simulink model "motor"  (Simulink 3.00)
libraries: mathlib x62, logiclib x16, reglib x10, execlib x6, genlib x6, anallib x4, arclib x1

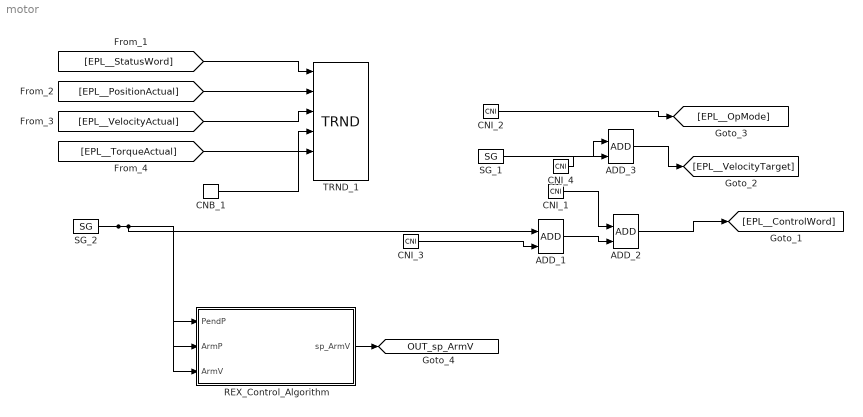
== system motor ==
  ADD_1 : mathlib/ADD
  ADD_2 : mathlib/ADD
  ADD_3 : mathlib/ADD
  CNB_1 : mathlib/CNB  YCN=on
  CNI_1 : mathlib/CNI  icn=15
  CNI_2 : mathlib/CNI  icn=3
  CNI_3 : mathlib/CNI  icn=64
  CNI_4 : mathlib/CNI  icn=0
  REX_Control_Algorithm : Subsystem  TreatAsAtomicUnit=on  SystemSampleTime=0.003
      mask Type: REX sequence
  SG_1 : genlib/SG  isig=1: SINE  amp=3000  freq=0.05  phase=0  ifrunit=1: Hz  iphunit=1: degree
  SG_2 : genlib/SG  isig=2: SQUARE  amp=64  freq=0.1  phase=0  ifrunit=1: Hz  iphunit=1: degree
  TRND_1 : arclib/TRND  n=4  l=1000  btype=8: Double  ptype1=1: Store  ptype2=1: Store  ptype3=1: Store  ptype4=1: Store  pfac=1  afac=0  arc=0  id=1  Title=Trend Title
  tag scope: OUT_sp_ArmV=global
  wires:
  ADD_1/1 -> ADD_2/2
  ADD_2/1 -> [EPL__ControlWord]
  ADD_3/1 -> [EPL__VelocityTarget]
  CNB_1/1 -> TRND_1/5
  CNI_1/1 -> ADD_2/1
  CNI_2/1 -> [EPL__OpMode]
  CNI_3/1 -> ADD_1/2
  CNI_4/1 -> ADD_3/2
  [EPL__StatusWord] -> TRND_1/1
  [EPL__PositionActual] -> TRND_1/2
  [EPL__VelocityActual] -> TRND_1/3
  [EPL__TorqueActual] -> TRND_1/4
  REX_Control_Algorithm/1(sp_ArmV) -> [OUT_sp_ArmV]
  SG_1/1 -> ADD_3/1
  SG_2/1 -> REX_Control_Algorithm/1(PendP), REX_Control_Algorithm/2(ArmP), ADD_1/1, REX_Control_Algorithm/3(ArmV)

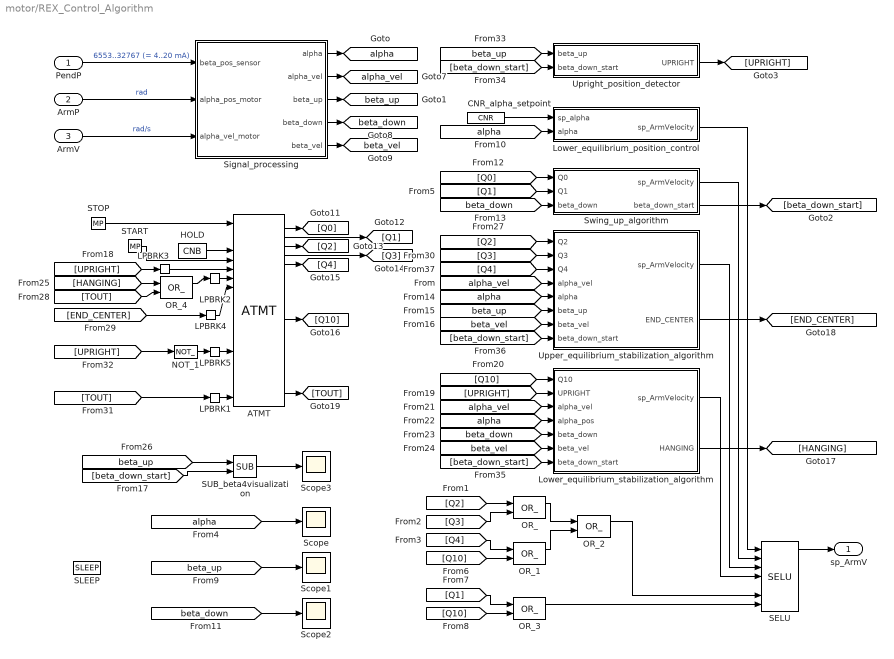
== system motor/REX_Control_Algorithm ==
  PendP : Inport  Port=1
  ArmP : Inport  Port=2
  ArmV : Inport  Port=3
  ATMT : logiclib/ATMT  SystemSampleTime=-1  morestps=off  ntr=10  STT=[0 0 1;1 1 2;1 15 0;2 3 3;3 15 4;4 15 10;10 2 0;2 10 0;3 10 0;4 10 0]  touts=[100 1 20 10 10 0 0 0 0 0 5 0 0 0 0 0]
  CNR_alpha_setpoint : mathlib/CNR  SystemSampleTime=-1  ycn=0
  HOLD : mathlib/CNB  SystemSampleTime=-1  YCN=off
  LPBRK{1..5} (5 alike) : execlib/LPBRK
  Lower_equilibrium_position_control : Subsystem
      mask Type: REX sequence
  Lower_equilibrium_stabilization_algorithm : Subsystem
      mask Type: REX sequence
  NOT_1 : logiclib/NOT_  SystemSampleTime=-1
  OR_{,1..4} (5 alike) : logiclib/OR_  SystemSampleTime=-1
  SELU : reglib/SELU  SystemSampleTime=-1  BINF=on
  SLEEP : execlib/SLEEP  SystemSampleTime=-1  ts=0.01
  START : genlib/MP  SystemSampleTime=-1  pwidth=0.01  BSTATE=off  RPTF=off
  STOP : genlib/MP  SystemSampleTime=-1  pwidth=0.01  BSTATE=off  RPTF=off
  SUB_beta4visualization : mathlib/SUB  SystemSampleTime=-1
  Scope{,1..3} (4 alike) : Scope
      Scope settings: TimeRange=60  YMin=-4  YMax=2
      Scope1 settings: TimeRange=60  YMin=-4  YMax=4
      Scope2 settings: YMin=2.97087  YMax=2.97104  SaveName=ScopeData2
      Scope3 settings: YMin=0  YMax=3.25  SaveName=ScopeData4
  Signal_processing : Subsystem
      mask Type: REX sequence
  Swing_up_algorithm : Subsystem
      mask Type: REX sequence
  Upper_equilibrium_stabilization_algorithm : Subsystem
      mask Type: REX sequence
  Upright_position_detector : Subsystem
      mask Type: REX sequence
  sp_ArmV : Outport  Port=1
  tag scope: alpha=global, alpha_vel=global, beta_down=global, beta_up=global, beta_vel=global
  wires:
  ATMT/1 -> [Q0]
  ATMT/2 -> [Q1]
  ATMT/3 -> [Q2]
  ATMT/4 -> [Q3]
  ATMT/5 -> [Q4]
  ATMT/11 -> [Q10]
  ATMT/19 -> [TOUT]
  ArmP/1 -> Signal_processing/2(alpha_pos_motor)  "rad"
  ArmV/1 -> Signal_processing/3(alpha_vel_motor)  "rad/s"
  CNR_alpha_setpoint/1 -> Lower_equilibrium_position_control/1(sp_alpha)
  [alpha_vel] -> Upper_equilibrium_stabilization_algorithm/4(alpha_vel)
  [Q2] -> OR_/1
  [alpha] -> Lower_equilibrium_position_control/2(alpha)
  [beta_down] -> Scope2/1
  [Q0] -> Swing_up_algorithm/1(Q0)
  [beta_down] -> Swing_up_algorithm/3(beta_down)
  [alpha] -> Upper_equilibrium_stabilization_algorithm/5(alpha)
  [beta_up] -> Upper_equilibrium_stabilization_algorithm/6(beta_up)
  [beta_vel] -> Upper_equilibrium_stabilization_algorithm/7(beta_vel)
  [beta_down_start] -> SUB_beta4visualization/2
  [UPRIGHT] -> LPBRK3/1
  [UPRIGHT] -> Lower_equilibrium_stabilization_algorithm/2(UPRIGHT)
  [Q3] -> OR_/2
  [Q10] -> Lower_equilibrium_stabilization_algorithm/1(Q10)
  [alpha_vel] -> Lower_equilibrium_stabilization_algorithm/3(alpha_vel)
  [alpha] -> Lower_equilibrium_stabilization_algorithm/4(alpha_pos)
  [beta_down] -> Lower_equilibrium_stabilization_algorithm/5(beta_down)
  [beta_vel] -> Lower_equilibrium_stabilization_algorithm/6(beta_vel)
  [HANGING] -> OR_4/1
  [beta_up] -> SUB_beta4visualization/1
  [Q2] -> Upper_equilibrium_stabilization_algorithm/1(Q2)
  [TOUT] -> OR_4/2
  [END_CENTER] -> LPBRK4/1
  [Q4] -> OR_1/1
  [Q3] -> Upper_equilibrium_stabilization_algorithm/2(Q3)
  [TOUT] -> LPBRK1/1
  [UPRIGHT] -> NOT_1/1
  [beta_up] -> Upright_position_detector/1(beta_up)
  [beta_down_start] -> Upright_position_detector/2(beta_down_start)
  [beta_down_start] -> Lower_equilibrium_stabilization_algorithm/7(beta_down_start)
  [beta_down_start] -> Upper_equilibrium_stabilization_algorithm/8(beta_down_start)
  [Q4] -> Upper_equilibrium_stabilization_algorithm/3(Q4)
  [alpha] -> Scope/1
  [Q1] -> Swing_up_algorithm/2(Q1)
  [Q10] -> OR_1/2
  [Q1] -> OR_3/1
  [Q10] -> OR_3/2
  [beta_up] -> Scope1/1
  HOLD/1 -> ATMT/4
  LPBRK1/1 -> ATMT/20
  LPBRK2/1 -> ATMT/7
  LPBRK3/1 -> ATMT/6
  LPBRK4/1 -> ATMT/8
  LPBRK5/1 -> ATMT/15
  Lower_equilibrium_position_control/1(sp_ArmVelocity) -> SELU/1
  Lower_equilibrium_stabilization_algorithm/1(sp_ArmVelocity) -> SELU/4
  Lower_equilibrium_stabilization_algorithm/2(HANGING) -> [HANGING]
  NOT_1/1 -> LPBRK5/1
  OR_/1 -> OR_2/1
  OR_1/1 -> OR_2/2
  OR_2/1 -> SELU/6
  OR_3/1 -> SELU/7
  OR_4/1 -> LPBRK2/1
  PendP/1 -> Signal_processing/1(beta_pos_sensor)  "6553..32767 (= 4..20 mA)"
  SELU/1 -> sp_ArmV/1
  START/1 -> ATMT/5
  STOP/1 -> ATMT/1
  SUB_beta4visualization/1 -> Scope3/1
  Signal_processing/1(alpha) -> [alpha]
  Signal_processing/2(alpha_vel) -> [alpha_vel]
  Signal_processing/3(beta_up) -> [beta_up]
  Signal_processing/4(beta_down) -> [beta_down]
  Signal_processing/5(beta_vel) -> [beta_vel]
  Swing_up_algorithm/1(sp_ArmVelocity) -> SELU/2
  Swing_up_algorithm/2(beta_down_start) -> [beta_down_start]
  Upper_equilibrium_stabilization_algorithm/1(sp_ArmVelocity) -> SELU/3
  Upper_equilibrium_stabilization_algorithm/2(END_CENTER) -> [END_CENTER]
  Upright_position_detector/1(UPRIGHT) -> [UPRIGHT]

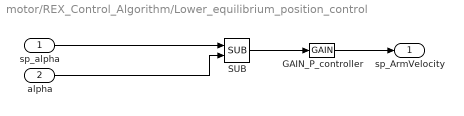
== system motor/REX_Control_Algorithm/Lower_equilibrium_position_control ==
  sp_alpha : Inport  Port=1
  alpha : Inport  Port=2
  GAIN_P_controller : mathlib/GAIN  SystemSampleTime=-1  k=2
  SUB : mathlib/SUB  SystemSampleTime=-1
  sp_ArmVelocity : Outport  Port=1
  wires:
  GAIN_P_controller/1 -> sp_ArmVelocity/1
  SUB/1 -> GAIN_P_controller/1
  alpha/1 -> SUB/2
  sp_alpha/1 -> SUB/1

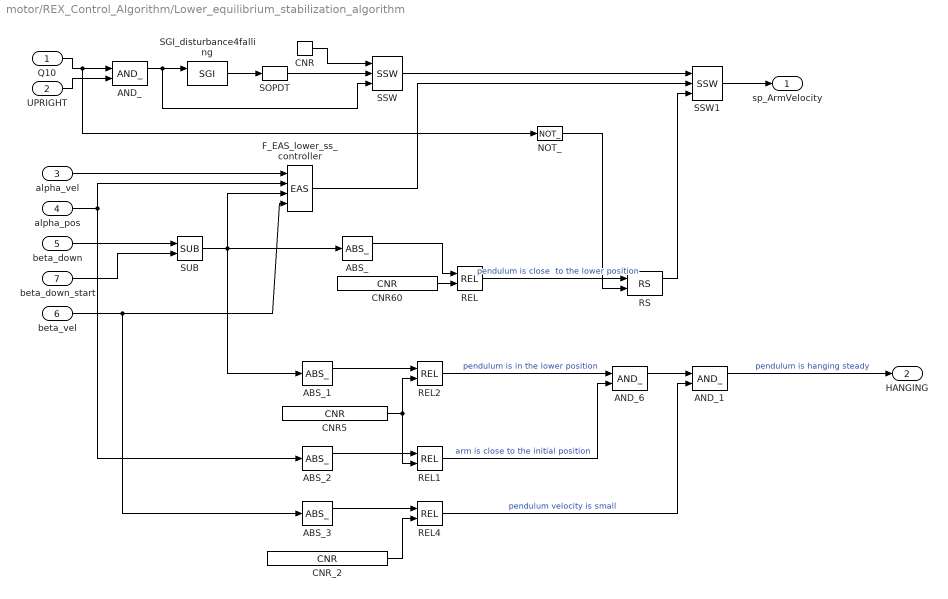
== system motor/REX_Control_Algorithm/Lower_equilibrium_stabilization_algorithm ==
  Q10 : Inport  Port=1
  UPRIGHT : Inport  Port=2
  alpha_vel : Inport  Port=3
  alpha_pos : Inport  Port=4
  beta_down : Inport  Port=5  OutDataType=sfix(16)  OutScaling=2^0
  beta_vel : Inport  Port=6  OutDataType=sfix(16)  OutScaling=2^0
  beta_down_start : Inport  Port=7  OutDataType=sfix(16)  OutScaling=2^0
  ABS_{,1..3} (4 alike) : mathlib/ABS_  SystemSampleTime=-1
  AND_ : logiclib/AND_  SystemSampleTime=-1
  AND_1 : logiclib/AND_  SystemSampleTime=-1
  AND_6 : logiclib/AND_  SystemSampleTime=-1
  CNR : mathlib/CNR  SystemSampleTime=-1  ycn=0
  CNR5 : mathlib/CNR  SystemSampleTime=-1  ycn=0.087266462599716
  CNR60 : mathlib/CNR  SystemSampleTime=-1  ycn=0.5
  CNR_2 : mathlib/CNR  SystemSampleTime=-1  ycn=0.0017453292519943
  F_EAS_lower_ss_controller : mathlib/EAS  SystemSampleTime=-1  a=6.12354219E-001  b=-4.25163230E-001  c=-2.53804417E+000  d=-3.30908089E-001  y0=0
  NOT_ : logiclib/NOT_  SystemSampleTime=-1
  REL{,1..2,4} (4 alike) : mathlib/REL  SystemSampleTime=-1  irel=3: less than (<)
  RS : logiclib/RS  SystemSampleTime=-1
  SGI_disturbance4falling : genlib/SGI  SystemSampleTime=-1  isig=4: RANDOM  amp=1  freq=1  phase=0  ifrunit=1: Hz  iphunit=1: degree
  SOPDT : reglib/SOPDT  SystemSampleTime=-1  itf=2: Real poles  k0=1  tau=0  tau1=0.1  tau2=0.2  om=1  xi=1  pb0=1  pb1=1  pa0=1  pa1=1  del=0
  SSW : reglib/SSW  SystemSampleTime=-1
  SSW1 : reglib/SSW  SystemSampleTime=-1
  SUB : mathlib/SUB  SystemSampleTime=-1
  sp_ArmVelocity : Outport  Port=1
  HANGING : Outport  Port=2
  wires:
  ABS_/1 -> REL/1
  ABS_1/1 -> REL2/1
  ABS_2/1 -> REL1/1
  ABS_3/1 -> REL4/1
  AND_/1 -> SGI_disturbance4falling/1, SSW/3
  AND_1/1 -> HANGING/1  "pendulum is hanging steady"
  AND_6/1 -> AND_1/1
  CNR/1 -> SSW/1
  CNR5/1 -> REL1/2, REL2/2
  CNR60/1 -> REL/2
  CNR_2/1 -> REL4/2
  F_EAS_lower_ss_controller/1 -> SSW1/2
  NOT_/1 -> RS/2
  Q10/1 -> AND_/1, NOT_/1
  REL/1 -> RS/1  "pendulum is close  to the lower position"
  REL1/1 -> AND_6/2  "arm is close to the initial position"
  REL2/1 -> AND_6/1  "pendulum is in the lower position"
  REL4/1 -> AND_1/2  "pendulum velocity is small"
  RS/1 -> SSW1/3
  SGI_disturbance4falling/1 -> SOPDT/1
  SOPDT/1 -> SSW/2
  SSW/1 -> SSW1/1
  SSW1/1 -> sp_ArmVelocity/1
  SUB/1 -> ABS_/1, ABS_1/1, F_EAS_lower_ss_controller/3
  UPRIGHT/1 -> AND_/2
  alpha_pos/1 -> ABS_2/1, F_EAS_lower_ss_controller/2
  alpha_vel/1 -> F_EAS_lower_ss_controller/1
  beta_down/1 -> SUB/1
  beta_down_start/1 -> SUB/2
  beta_vel/1 -> ABS_3/1, F_EAS_lower_ss_controller/4

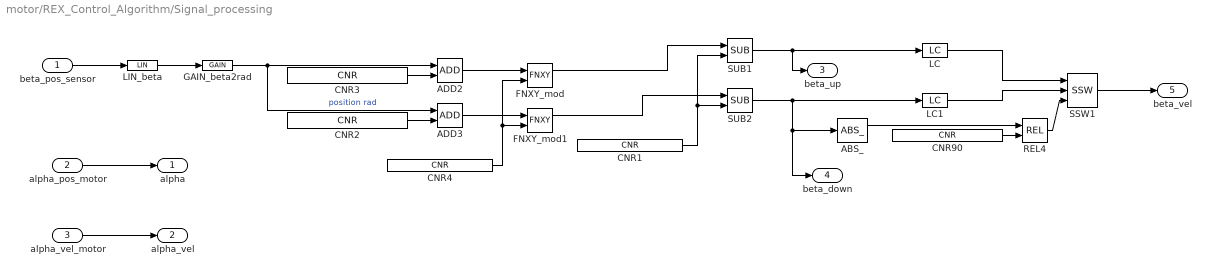
== system motor/REX_Control_Algorithm/Signal_processing ==
  beta_pos_sensor : Inport  Port=1
  alpha_pos_motor : Inport  Port=2
  alpha_vel_motor : Inport  Port=3
  ABS_ : mathlib/ABS_  SystemSampleTime=-1
  ADD2 : mathlib/ADD  SystemSampleTime=-1
  ADD3 : mathlib/ADD  SystemSampleTime=-1
  CNR1 : mathlib/CNR  SystemSampleTime=-1  ycn=3.14159265358979
  CNR2 : mathlib/CNR  SystemSampleTime=-1  ycn=4.71238898038469
  CNR3 : mathlib/CNR  SystemSampleTime=-1  ycn=7.853981633974483
  CNR4 : mathlib/CNR  SystemSampleTime=-1  ycn=6.283185307179586
  CNR90 : mathlib/CNR  SystemSampleTime=-1  ycn=1.570796326794897
  FNXY_mod : mathlib/FNXY  SystemSampleTime=-1  ifn=2: fmod  yerr=0.0
  FNXY_mod1 : mathlib/FNXY  SystemSampleTime=-1  ifn=2: fmod  yerr=0.0
  GAIN_beta2rad : mathlib/GAIN  SystemSampleTime=-1  k=0.0175
  LC : reglib/LC  SystemSampleTime=-1  td=1  nd=30  ISSF=off
  LC1 : reglib/LC  SystemSampleTime=-1  td=1  nd=30  ISSF=off
  LIN_beta : mathlib/LIN  SystemSampleTime=-1  u1=6553  y1=5  u2=32767  y2=355
  REL4 : mathlib/REL  SystemSampleTime=-1  irel=3: less than (<)
  SSW1 : reglib/SSW  SystemSampleTime=-1
  SUB1 : mathlib/SUB  SystemSampleTime=-1
  SUB2 : mathlib/SUB  SystemSampleTime=-1
  alpha : Outport  Port=1
  alpha_vel : Outport  Port=2
  beta_up : Outport  Port=3
  beta_down : Outport  Port=4
  beta_vel : Outport  Port=5
  wires:
  ABS_/1 -> REL4/1
  ADD2/1 -> FNXY_mod/1
  ADD3/1 -> FNXY_mod1/1
  CNR1/1 -> SUB1/2, SUB2/2
  CNR2/1 -> ADD3/2
  CNR3/1 -> ADD2/2
  CNR4/1 -> FNXY_mod/2, FNXY_mod1/2
  CNR90/1 -> REL4/2
  FNXY_mod/1 -> SUB1/1
  FNXY_mod1/1 -> SUB2/1
  GAIN_beta2rad/1 -> ADD2/1, ADD3/1  "position rad"
  LC/1 -> SSW1/1
  LC1/1 -> SSW1/2
  LIN_beta/1 -> GAIN_beta2rad/1
  REL4/1 -> SSW1/3
  SSW1/1 -> beta_vel/1
  SUB1/1 -> LC/1, beta_up/1
  SUB2/1 -> ABS_/1, beta_down/1, LC1/1
  alpha_pos_motor/1 -> alpha/1
  alpha_vel_motor/1 -> alpha_vel/1
  beta_pos_sensor/1 -> LIN_beta/1

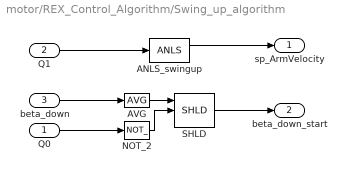
== system motor/REX_Control_Algorithm/Swing_up_algorithm ==
  Q0 : Inport  Port=1
  Q1 : Inport  Port=2
  beta_down : Inport  Port=3  OutDataType=sfix(16)  OutScaling=2^0
  ANLS_swingup : genlib/ANLS  SystemSampleTime=-1  y0=-10  t1=0.21  y1=-10  t2=0.21  y2=10  t3=1  y3=10  t4=1  y4=0  RPT=off
  AVG : anallib/AVG  SystemSampleTime=-1  n=100
  NOT_2 : logiclib/NOT_  SystemSampleTime=-1
  SHLD : anallib/SHLD  SystemSampleTime=-1  y0=0
  sp_ArmVelocity : Outport  Port=1
  beta_down_start : Outport  Port=2
  wires:
  ANLS_swingup/1 -> sp_ArmVelocity/1
  AVG/1 -> SHLD/1
  NOT_2/1 -> SHLD/2
  Q0/1 -> NOT_2/1
  Q1/1 -> ANLS_swingup/1
  SHLD/1 -> beta_down_start/1
  beta_down/1 -> AVG/1

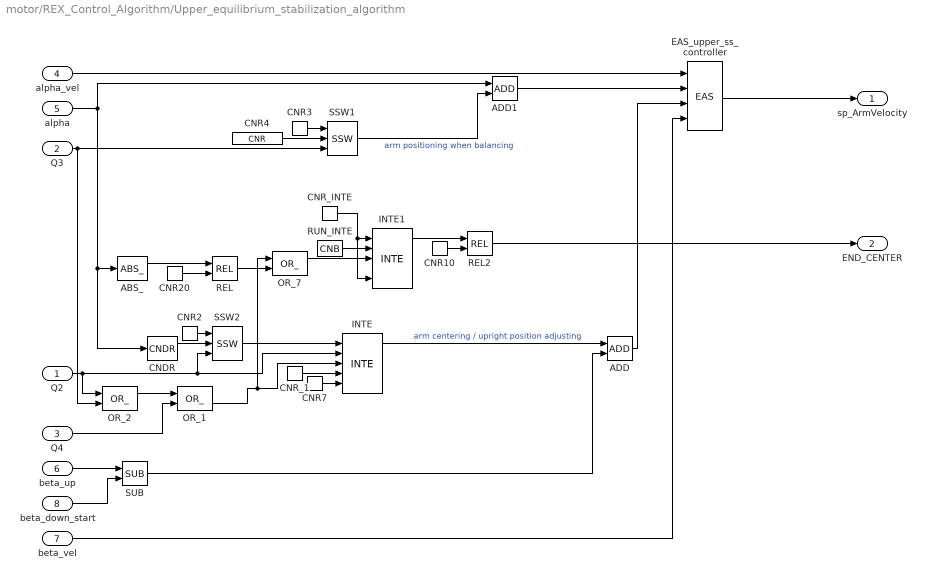
== system motor/REX_Control_Algorithm/Upper_equilibrium_stabilization_algorithm ==
  Q2 : Inport  Port=1
  Q3 : Inport  Port=2
  Q4 : Inport  Port=3
  alpha_vel : Inport  Port=4
  alpha : Inport  Port=5
  beta_up : Inport  Port=6  OutDataType=sfix(16)  OutScaling=2^0
  beta_vel : Inport  Port=7  OutDataType=sfix(16)  OutScaling=2^0
  beta_down_start : Inport  Port=8  OutDataType=sfix(16)  OutScaling=2^0
  ABS_ : mathlib/ABS_  SystemSampleTime=-1
  ADD : mathlib/ADD  SystemSampleTime=-1
  ADD1 : mathlib/ADD  SystemSampleTime=-1
  CNDR : reglib/CNDR  SystemSampleTime=-1  n=6  SATF=on  up=[-1.5708 -0.7854 -0.0523 0.0523 0.7854 1.5708]  yp=[-0.12 -0.04 0 0 0.04 0.12]
  CNR10 : mathlib/CNR  SystemSampleTime=-1  ycn=20
  CNR2 : mathlib/CNR  SystemSampleTime=-1  ycn=0
  CNR20 : mathlib/CNR  SystemSampleTime=-1  ycn=0.349065850398866
  CNR3 : mathlib/CNR  SystemSampleTime=-1  ycn=0
  CNR4 : mathlib/CNR  SystemSampleTime=-1  ycn=3.1415
  CNR7 : mathlib/CNR  SystemSampleTime=-1  ycn=20
  CNR_1 : mathlib/CNR  SystemSampleTime=-1  ycn=0
  CNR_INTE : mathlib/CNR  SystemSampleTime=-1  ycn=1
  EAS_upper_ss_controller : mathlib/EAS  SystemSampleTime=-1  a=1.129252325  b=0.9969568362e-1  c=3.607536576  d=.5522734341  y0=0
  INTE : anallib/INTE  SystemSampleTime=-1  ymin=-1  ymax=1
  INTE1 : anallib/INTE  SystemSampleTime=-1  ymin=0  ymax=30
  OR_1 : logiclib/OR_  SystemSampleTime=-1
  OR_2 : logiclib/OR_  SystemSampleTime=-1
  OR_7 : logiclib/OR_  SystemSampleTime=-1
  REL : mathlib/REL  SystemSampleTime=-1  irel=6: greater or equal (>=)
  REL2 : mathlib/REL  SystemSampleTime=-1  irel=6: greater or equal (>=)
  RUN_INTE : mathlib/CNB  SystemSampleTime=-1  YCN=on
  SSW1 : reglib/SSW  SystemSampleTime=-1
  SSW2 : reglib/SSW  SystemSampleTime=-1
  SUB : mathlib/SUB  SystemSampleTime=-1
  sp_ArmVelocity : Outport  Port=1
  END_CENTER : Outport  Port=2
  wires:
  ABS_/1 -> REL/1
  ADD/1 -> EAS_upper_ss_controller/3
  ADD1/1 -> EAS_upper_ss_controller/2
  CNDR/1 -> SSW2/2
  CNR10/1 -> REL2/2
  CNR2/1 -> SSW2/1
  CNR20/1 -> REL/2
  CNR3/1 -> SSW1/1
  CNR4/1 -> SSW1/2
  CNR7/1 -> INTE/5
  CNR_1/1 -> INTE/4
  CNR_INTE/1 -> INTE1/1, INTE1/5
  EAS_upper_ss_controller/1 -> sp_ArmVelocity/1
  INTE/1 -> ADD/1  "arm centering / upright position adjusting"
  INTE1/1 -> REL2/1
  OR_1/2 -> INTE/3, OR_7/1
  OR_2/1 -> OR_1/1
  OR_7/1 -> INTE1/3
  Q2/1 -> INTE/2, SSW2/3, OR_2/1
  Q3/1 -> OR_2/2, SSW1/3
  Q4/1 -> OR_1/2
  REL/1 -> OR_7/2
  REL2/1 -> END_CENTER/1
  RUN_INTE/1 -> INTE1/2
  SSW1/1 -> ADD1/2  "arm positioning when balancing"
  SSW2/1 -> INTE/1
  SUB/1 -> ADD/2
  alpha/1 -> ADD1/1, ABS_/1, CNDR/1
  alpha_vel/1 -> EAS_upper_ss_controller/1
  beta_down_start/1 -> SUB/2
  beta_up/1 -> SUB/1
  beta_vel/1 -> EAS_upper_ss_controller/4

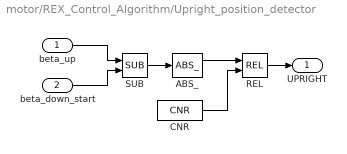
== system motor/REX_Control_Algorithm/Upright_position_detector ==
  beta_up : Inport  Port=1
  beta_down_start : Inport  Port=2
  ABS_ : mathlib/ABS_  SystemSampleTime=-1
  CNR : mathlib/CNR  SystemSampleTime=-1  ycn=0.9
  REL : mathlib/REL  SystemSampleTime=-1  irel=3: less than (<)
  SUB : mathlib/SUB  SystemSampleTime=-1
  UPRIGHT : Outport  Port=1
  wires:
  ABS_/1 -> REL/1
  CNR/1 -> REL/2
  REL/1 -> UPRIGHT/1
  SUB/1 -> ABS_/1
  beta_down_start/1 -> SUB/2
  beta_up/1 -> SUB/1
